simulink model "simulate_sensors"  (R2025a)
settings: Solver=FixedStepAuto  StartTime=0.0  StopTime=50  FixedStep=dt_ekf  RelTol=1e-3
values from neighbouring files (symbols this model uses):
  dt_ekf = 1/1000    (= 0.001)    [ekf_2d_simulink.m]    (also in ekf_2d_tutorial.m; ekf_3d.m)
  dt_gps = 1/5    (= 0.2)    [ekf_2d_simulink.m]    (also in ekf_2d_tutorial.m; ekf_3d.m = 1)
undefined symbols (not defined in the file or in its folder): fractalcoef
libraries: simulink x3, mspsensorlib x2, simulink_extras x2
settings Model: Creator=jonno  LastModifiedBy=jonno

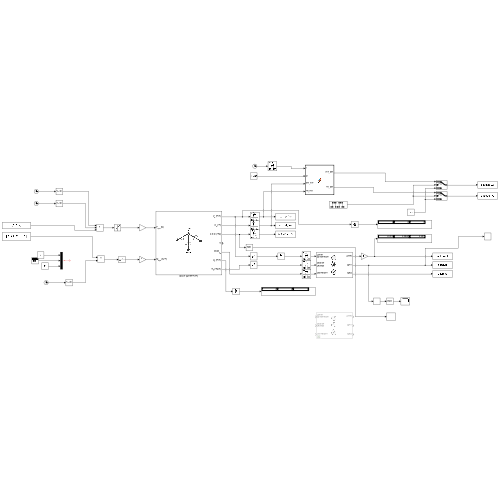
[thumbnail: Simulink's stored preview of the top-level diagram]
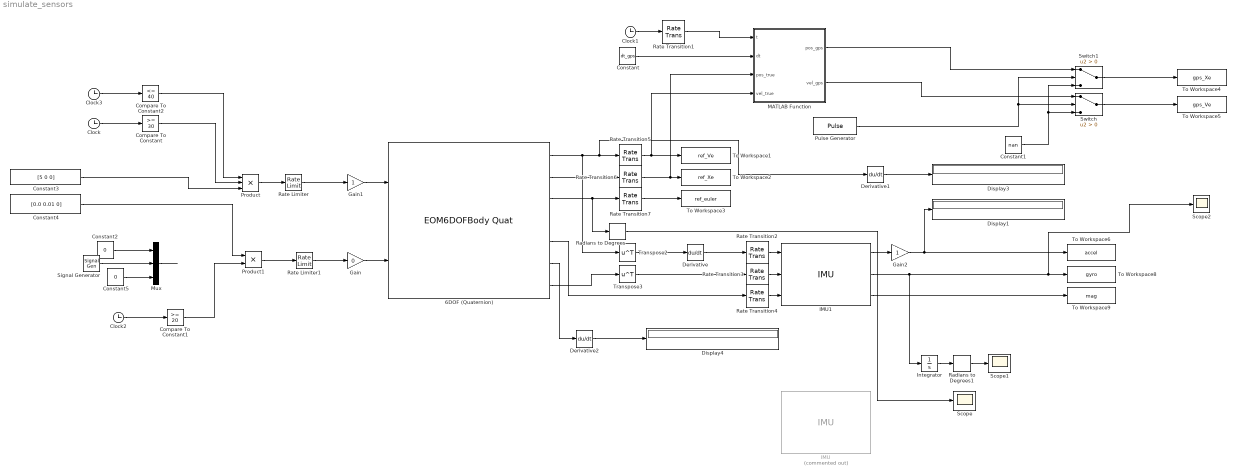
== system simulate_sensors ==
  6DOF (Quaternion) : EOM6DOFBodyQuat  eul_0=[deg2rad(0) deg2rad(0) deg2rad(0)]
  Clock{,1..3} (4 alike) : Clock
  Compare To Constant : simulink/Logic and Bit Operations/Compare To Constant  relop=>=  const=30  OutDataTypeStr=boolean
  Compare To Constant1 : simulink/Logic and Bit Operations/Compare To Constant  relop=>=  const=20  OutDataTypeStr=boolean
  Compare To Constant2 : simulink/Logic and Bit Operations/Compare To Constant  relop=<=  const=40  OutDataTypeStr=boolean
  Constant : Constant  Value=dt_gps
  Constant1 : Constant  Value=nan
  Constant2 : Constant  Value=0
  Constant3 : Constant  Value=[5 0 0]
  Constant4 : Constant  Value=[0.0 0.01 0]
  Constant5 : Constant  Value=0
  Derivative : Derivative
  Derivative1 : Derivative
  Derivative2 : Derivative
  Display1 : Display
  Display3 : Display
  Display4 : Display
  Gain : Gain  Gain=0
  Gain1 : Gain
  Gain2 : Gain
  IMU : mspsensorlib/IMU  Commented=on  DispRefFrame=NED  TemperaturePort=off  Temperature=25  MagneticFieldPort=off  MagneticFieldNED=[ 27.5550, -2.4169, -16.0849 ]  MagneticFieldENU=[ -2.4169, 27.5550, 16.0849 ]  SeedDouble=67  SimulateUsing=Code generation  AccelParamsMeasurementRange=16*9.81  AccelParamsResolution=((0.732)/1000)*9.81  AccelParamsConstantBias=[0 0.0 0.0]  AccelParamsAxesMisalignment=[0 0 0]  AccelParamsNoiseDensity=[0 0 0]  AccelParamsBiasInstability=[0 0 0]  AccelParamsBiasInstabilityNumerator=fractalcoef().Numerator  AccelParamsBiasInstabilityDenominator=fractalcoef().Denominator  AccelParamsRandomWalk=[0 0 0]  AccelParamsNoiseType=double-sided  AccelParamsTemperatureBias=[0 0 0]  AccelParamsTemperatureScaleFactor=[0 0 0]  GyroParamsMeasurementRange=34.9066  GyroParamsResolution=0.0017453  GyroParamsConstantBias=[0 0 0]  GyroParamsAxesMisalignment=0  GyroParamsAccelerationBias=[0 0 0]  GyroParamsNoiseDensity=[2.9e-4 2.9e-4 2.9e-4]  GyroParamsBiasInstability=[4.8e-5 4.8e-5 4.8e-5]  GyroParamsBiasInstabilityNumerator=fractalcoef().Numerator  GyroParamsBiasInstabilityDenominator=fractalcoef().Denominator  GyroParamsRandomWalk=[0 0 0]  GyroParamsNoiseType=double-sided  GyroParamsTemperatureBias=[0 0 0]  GyroParamsTemperatureScaleFactor=[0 0 0]  MagParamsMeasurementRange=800  MagParamsResolution=0.025  MagParamsConstantBias=0  MagParamsAxesMisalignment=[0 0 0]  MagParamsNoiseDensity=[0 0 0]  MagParamsBiasInstability=[0 0 0]  MagParamsBiasInstabilityNumerator=fractalcoef().Numerator  MagParamsBiasInstabilityDenominator=fractalcoef().Denominator  MagParamsRandomWalk=[0 0 0]  MagParamsNoiseType=double-sided  MagParamsTemperatureBias=[0 0 0]  MagParamsTemperatureScaleFactor=[0 0 0]
  IMU1 : mspsensorlib/IMU  DispRefFrame=NED  TemperaturePort=off  Temperature=25  MagneticFieldPort=off  MagneticFieldNED=[ 27.5550, -2.4169, -16.0849 ]  MagneticFieldENU=[ -2.4169, 27.5550, 16.0849 ]  SeedDouble=67  SimulateUsing=Code generation  AccelParamsMeasurementRange=16*9.81  AccelParamsResolution=((0.732)/1000)*9.81  AccelParamsConstantBias=[0 0.0 0.0]  AccelParamsAxesMisalignment=[0 0 0]  AccelParamsNoiseDensity=[3.9e-3 3.9e-3 3.9e-3].*1  AccelParamsBiasInstability=[5.0e-3 5.0e-3 5.0e-3].*1  AccelParamsBiasInstabilityNumerator=fractalcoef().Numerator  AccelParamsBiasInstabilityDenominator=fractalcoef().Denominator  AccelParamsRandomWalk=[0 0 0]  AccelParamsNoiseType=double-sided  AccelParamsTemperatureBias=[0 0 0]  AccelParamsTemperatureScaleFactor=[0 0 0]  GyroParamsMeasurementRange=34.9066  GyroParamsResolution=0.0017453  GyroParamsConstantBias=[1 1 0].*deg2rad(0.01)  GyroParamsAxesMisalignment=0  GyroParamsAccelerationBias=[0 0 0]  GyroParamsNoiseDensity=[3.0e-3 3.0e-3 3.0e-3]  GyroParamsBiasInstability=[4.8e-4 4.8e-4 4.8e-4]  GyroParamsBiasInstabilityNumerator=fractalcoef().Numerator  GyroParamsBiasInstabilityDenominator=fractalcoef().Denominator  GyroParamsRandomWalk=[0 0 0]  GyroParamsNoiseType=double-sided  GyroParamsTemperatureBias=[0 0 0]  GyroParamsTemperatureScaleFactor=[0 0 0]  MagParamsMeasurementRange=800  MagParamsResolution=0.025  MagParamsConstantBias=0  MagParamsAxesMisalignment=[0 0 0]  MagParamsNoiseDensity=[0.1 0.1 0.1]  MagParamsBiasInstability=[0 0 0]  MagParamsBiasInstabilityNumerator=fractalcoef().Numerator  MagParamsBiasInstabilityDenominator=fractalcoef().Denominator  MagParamsRandomWalk=[0 0 0]  MagParamsNoiseType=double-sided  MagParamsTemperatureBias=[0 0 0]  MagParamsTemperatureScaleFactor=[0 0 0]
  Integrator : Integrator
  MATLAB Function : MATLAB Function  TreatAsAtomicUnit=on
  Mux : Mux  Inputs=3
  Product : Product  Inputs=3
  Product1 : Product
  Pulse Generator : DiscretePulseGenerator  Period=dt_gps/dt_ekf  SampleTime=dt_ekf
  Radians to Degrees : simulink_extras/Transformations/Radians to Degrees
  Radians to Degrees1 : simulink_extras/Transformations/Radians to Degrees
  Rate Limiter : RateLimiter  SampleTimeMode=inherited
  Rate Limiter1 : RateLimiter  RisingSlewLimit=0.2  FallingSlewLimit=-0.2  SampleTimeMode=inherited
  Rate Transition{1..7} (7 alike) : RateTransition  OutPortSampleTime=dt_ekf
  Scope : Scope
      settings: ActiveDisplayYMinimum=-10.419736242536136  ActiveDisplayYMaximum=86.999248894017285
  Scope1 : Scope
      settings: ActiveDisplayYMinimum=-17.490435795984297  ActiveDisplayYMaximum=92.586437441472384
  Scope2 : Scope
      settings: ActiveDisplayYMinimum=-0.75312484070589725  ActiveDisplayYMaximum=0.83015131565189693  DataLoggingVariableName=ScopeData2
  Signal Generator : SignalGenerator  Amplitude=2*pi/180  Frequency=0.2
  Switch : Switch  Criteria=u2 > Threshold  SaturateOnIntegerOverflow=off  InputSameDT=off
  Switch1 : Switch  Criteria=u2 > Threshold  SaturateOnIntegerOverflow=off  InputSameDT=off
  To Workspace1 : ToWorkspace  VariableName=ref_Ve  SaveFormat=Timeseries  SampleTime=-1
  To Workspace2 : ToWorkspace  VariableName=ref_Xe  SaveFormat=Timeseries  SampleTime=-1
  To Workspace3 : ToWorkspace  VariableName=ref_euler  SaveFormat=Timeseries  SampleTime=-1
  To Workspace4 : ToWorkspace  VariableName=gps_Xe  SaveFormat=Timeseries  SampleTime=-1
  To Workspace5 : ToWorkspace  VariableName=gps_Ve  SaveFormat=Timeseries  SampleTime=-1
  To Workspace6 : ToWorkspace  VariableName=accel  SaveFormat=Timeseries  SampleTime=-1
  To Workspace8 : ToWorkspace  VariableName=gyro  SaveFormat=Timeseries  SampleTime=-1
  To Workspace9 : ToWorkspace  VariableName=mag  SaveFormat=Timeseries  SampleTime=-1
  Transpose2 : Math  Operator=transpose
  Transpose3 : Math  Operator=transpose
  wires:
  Derivative/1 -> Rate Transition2/1
  6DOF (Quaternion)/7 -> Transpose3/1
  Transpose3/1 -> Rate Transition3/1
  IMU1/2 -> Integrator/1, Scope2/1, To Workspace8/1
  Rate Transition4/1 -> IMU1/3
  Transpose2/1 -> Derivative/1
  Rate Transition2/1 -> IMU1/1
  6DOF (Quaternion)/2 -> Rate Transition6/1
  Rate Transition3/1 -> IMU1/2
  Pulse Generator/1 -> Switch/2, Switch1/2
  IMU1/3 -> To Workspace9/1
  Constant1/1 -> Switch1/3, Switch/3
  6DOF (Quaternion)/5 -> Rate Transition4/1
  Switch1/1 -> To Workspace4/1
  Switch/1 -> To Workspace5/1
  6DOF (Quaternion)/3 -> Radians to Degrees/1, Rate Transition7/1
  Rate Transition7/1 -> To Workspace3/1
  IMU1/1 -> Gain2/1
  Gain/1 -> 6DOF (Quaternion)/2
  Radians to Degrees/1 -> Scope/1
  Integrator/1 -> Radians to Degrees1/1
  Radians to Degrees1/1 -> Scope1/1
  Derivative1/1 -> Display3/1
  Derivative2/1 -> Display4/1
  6DOF (Quaternion)/6 -> Derivative2/1
  Gain2/1 -> Display1/1, To Workspace6/1
  6DOF (Quaternion)/1 -> Transpose2/1, Derivative1/1, Rate Transition5/1
  Gain1/1 -> 6DOF (Quaternion)/1
  Mux/1 -> ?
  Constant2/1 -> Mux/1
  Constant5/1 -> Mux/3
  Signal Generator/1 -> Mux/2
  Product/1 -> Rate Limiter/1
  Clock/1 -> Compare To Constant/1
  Rate Limiter1/1 -> Gain/1
  Product1/1 -> Rate Limiter1/1
  Constant4/1 -> Product1/1
  Constant3/1 -> Product/3
  Rate Transition6/1 -> MATLAB Function/3(pos_true), To Workspace2/1
  Rate Transition5/1 -> MATLAB Function/4(vel_true), To Workspace1/1
  Clock1/1 -> Rate Transition1/1
  Rate Transition1/1 -> MATLAB Function/1(t)
  Constant/1 -> MATLAB Function/2(dt)
  MATLAB Function/1(pos_gps) -> Switch1/1
  MATLAB Function/2(vel_gps) -> Switch/1
  Compare To Constant/1 -> Product/2
  Clock2/1 -> Compare To Constant1/1
  Compare To Constant1/1 -> Product1/2
  Clock3/1 -> Compare To Constant2/1
  Compare To Constant2/1 -> Product/1
  Rate Limiter/1 -> Gain1/1

== matlab function simulate_sensors/MATLAB Function ==
  data: t input; dt input; pos_true input; pos_gps output; vel_true input; vel_gps output
function [pos_gps, vel_gps] = fcn(t, dt, pos_true, vel_true)
% This function simulates a GPS sensor by adding noise and holding the
% signal to replicate a specific update rate.

% Sensor Characteristics
persistent last_t pos_meas vel_meas; % Stores the last measurement time and values
sample_time = dt; % GPS update period in seconds (1 Hz)
pos_std_dev = 5.0; % Standard deviation of position noise in meters
vel_std_dev = 0.5; % Standard deviation of velocity noise in m/s

% Initialize persistent variables if they are empty
if isempty(last_t)
    last_t = -sample_time;
    pos_meas = pos_true;
    vel_meas = vel_true;
end

% Get the current simulation time


% Check if it's time to take a new measurement
if (t - last_t) >= sample_time
    % Update the last measurement time
    last_t = t;
    
    % Add Gaussian noise to the true values to simulate a new reading
    pos_noise = pos_std_dev * randn(size(pos_true));
    vel_noise = vel_std_dev * randn(size(vel_true));
    
    pos_meas = pos_true + pos_noise;
    vel_meas = vel_true + vel_noise;
end

% Output the last recorded measurement (Zero-Order Hold)
pos_gps = pos_meas;
vel_gps = vel_meas;

end
